simulink model "auto_pilot_upl_20240129"  (R2022b)
settings: Solver=FixedStepAuto  StartTime=0.0  StopTime=Inf  FixedStep=0.001  RelTol=1e-3  EnableMultiTasking=on
InitFcn:
  | clear mex
model workspace (MAT data in the model file):
  worldsim_instance.endpoint_ip = '127.0.0.1'
  worldsim_instance.endpoint_port = 8080
values from neighbouring files (symbols this model uses):
  ACC_Adaptive_D = 0    [AutoPilot_parameters.m]    (also in ap_ini_param.mat; ap_initialModel.sldd = 0.0)
  ACC_Adaptive_I = 0    [AutoPilot_parameters.m]    (also in ap_ini_param.mat; ap_initialModel.sldd = 0.0)
  ACC_Adaptive_P = [5 7.5]    [AutoPilot_parameters.m]    (also in ap_ini_param.mat; ap_initialModel.sldd = 5.0 7.5)
  ACC_Classic_I = 5    [AutoPilot_parameters.m]    (also in ap_ini_param.mat; ap_initialModel.sldd = 5.0)
  ACC_Classic_P = 15    [AutoPilot_parameters.m]    (also in ap_ini_param.mat; ap_initialModel.sldd = 15.0)
  ACC_MaxBrake = 50    [AutoPilot_parameters.m]    (also in ap_ini_param.mat; ap_initialModel.sldd = 50.0)
  ACC_MaxThrottle = 130    [AutoPilot_parameters.m]    (also in ap_ini_param.mat = 80; ap_initialModel.sldd = 130.0)
  ACC_Module_Activity_Flag = 1    [AutoPilot_parameters.m]    (also in ap_ini_param.mat; ap_initialModel.sldd = 1.0)
  ACC_Ready_Speed = 30    [AutoPilot_parameters.m]    (also in ap_ini_param.mat; ap_initialModel.sldd = 30.0)
  ACC_SensorMaxDistance = 250    [AutoPilot_parameters.m]    (also in ap_ini_param.mat = 120; ap_initialModel.sldd = 250.0)
  ACC_Speed_Distance_control = 3    [AutoPilot_parameters.m]    (also in ap_ini_param.mat; ap_initialModel.sldd = 3.0)
  ACC_Speed_Distance_Gain = [0.1 0.15 0.2 0.25]    [AutoPilot_parameters.m]    (also in ap_ini_param.mat; ap_initialModel.sldd = 0.1 0.15 0.2 0.25)
  ADAS_Control_Mode = 1    [AutoPilot_parameters.m]    (also in ap_ini_param.mat; ap_initialModel.sldd = 1.0)
  AEB_Alarm_Freq = 5    [AutoPilot_parameters.m]    (also in ap_ini_param.mat; ap_initialModel.sldd = 5.0)
  AEB_Distance_To_Collision_Brake = 5    [AutoPilot_parameters.m]    (also in ap_ini_param.mat; ap_initialModel.sldd = 5.0)
  AEB_Freq_Hz = Sensor_Freq_worldsim/2    (= 25)    [AutoPilot_parameters.m]    (also in ap_ini_param.mat; ap_initialModel.sldd = 25.0)
  AEB_Gain = [1 1]    [AutoPilot_parameters.m]    (also in ap_ini_param.mat; ap_initialModel.sldd = 1.0 1.0)
  AEB_Gain_set = 60    [AutoPilot_parameters.m]    (also in ap_ini_param.mat; ap_initialModel.sldd = 60.0)
  AEB_Gain_set_mult = 0.03    [AutoPilot_parameters.m]    (also in ap_ini_param.mat; ap_initialModel.sldd)
  AEB_Max_Decel = [8 15]    [AutoPilot_parameters.m]    (also in ap_ini_param.mat; ap_initialModel.sldd = 8.0 15.0)
  AEB_Max_Speed = 150    [AutoPilot_parameters.m]    (also in ap_ini_param.mat = 100; ap_initialModel.sldd = 150.0)
  AEB_Min_Distance_at_Stop = 1    [AutoPilot_parameters.m]    (also in ap_ini_param.mat; ap_initialModel.sldd = 1.0)
  AEB_Module_Activity_Flag = 1    [AutoPilot_parameters.m]    (also in ap_ini_param.mat; ap_initialModel.sldd = 1.0)
  AEB_Pedestrian_type = 68    [AutoPilot_parameters.m]    (also in ap_ini_param.mat; ap_initialModel.sldd = 68.0)
  AEB_Steer_Max = 180    [AutoPilot_parameters.m]    (also in ap_ini_param.mat; ap_initialModel.sldd = 180.0)
  AP_Activity_Flag = 1    [AutoPilot_parameters.m]    (also in ap_ini_param.mat; ap_initialModel.sldd = 1.0)
  AP_D = [0.3 0.3]    [AutoPilot_parameters.m]    (also in ap_ini_param.mat; ap_initialModel.sldd = 0.3 0.3)
  AP_Dyn_Rate_Limiter_Gain = 0.1    [AutoPilot_parameters.m]    (also in ap_ini_param.mat; ap_initialModel.sldd)
  AP_Dyn_Rate_Limiter_Power = 10    [AutoPilot_parameters.m]    (also in ap_ini_param.mat; ap_initialModel.sldd = 10.0)
  AP_Error_Max = 3    [AutoPilot_parameters.m]    (also in ap_ini_param.mat; ap_initialModel.sldd = 3.0)
  AP_Freq_Hz = Sensor_Freq_worldsim    (= 50)    [AutoPilot_parameters.m]    (also in ap_ini_param.mat; ap_initialModel.sldd = 50.0)
  AP_I = [0.05 0.05]    [AutoPilot_parameters.m]    (also in ap_ini_param.mat; ap_initialModel.sldd = 0.05 0.05)
  AP_Max_Error_dydt_Disable = 0.5    [AutoPilot_parameters.m]    (also in ap_ini_param.mat; ap_initialModel.sldd)
  AP_On_Request_Time = 0.01    [AutoPilot_parameters.m]    (also in ap_ini_param.mat; ap_initialModel.sldd)
  AP_P = [0.2 0.2]    [AutoPilot_parameters.m]    (also in ap_ini_param.mat; ap_initialModel.sldd = 0.2 0.2)
  AP_Steer_Error_Max = 0.7    [AutoPilot_parameters.m]    (also in ap_ini_param.mat; ap_initialModel.sldd)
  AP_Steer_Rate_Max_radps = 1    [AutoPilot_parameters.m]    (also in ap_ini_param.mat; ap_initialModel.sldd = 1.0)
  AP_Transition_Rate = 0.5    [AutoPilot_parameters.m]    (also in ap_ini_param.mat; ap_initialModel.sldd)
  butter_a = [1 -1.9911142922 0.991153595869]    [ap_ini_param.mat]    (also in ap_initialModel.sldd = 1.0 -1.9911142922016536 0.99115359586893548)
  butter_b = [9.82591682048e-06 1.9651833641e-05 9.82591682048e-06]    [ap_ini_param.mat]    (also in ap_initialModel.sldd = 9.825916820482009E-6 1.9651833640964018E-5 9.825916820482009)
  Lane_Width = 3.7    [AutoPilot_parameters.m]    (also in ap_ini_param.mat; ap_initialModel.sldd)
  No_Target_Display_Value = 0    [AutoPilot_parameters.m]    (also in ap_ini_param.mat; ap_initialModel.sldd = 0.0)
  radar_source = 2    [AutoPilot_parameters.m]    (also in ap_ini_param.mat; ap_initialModel.sldd = 2.0)
  Sensor_Freq_worldsim = 50    [AutoPilot_parameters.m]    (also in ap_ini_param.mat; ap_initialModel.sldd = 50.0; launcher.m)
  stop_number_collisions = 10.0    [ap_initialModel.sldd]    (also in launcher.m = 10)
  stop_speed = 0.001    [ap_initialModel.sldd]    (also in launcher.m)
  stop_time = 12.0    [ap_initialModel.sldd]    (also in launcher.m = 12)
  vehicle_width = 2.2    [AutoPilot_parameters.m]    (also in ap_ini_param.mat = 1.86; ap_initialModel.sldd)
undefined symbols (not defined in the file or in its folder): blockPlatform, light_brake_center, light_brake_left, light_brake_right
libraries: simulink x82, simwbSfunlib x32, viworldsim_lib x5, slpidlib x4, simwbUDPBlocklib x1
(part 1 of 4)
settings Model: Creator=mcava  LastModifiedBy=pumpaipa
settings SolverCC: AlgebraicLoopSolver=TrustRegion  AutoInsertRateTranBlk=on
settings DataIOCC: LimitDataPoints=on  SaveFormat=Array  ReturnWorkspaceOutputs=off  SignalLoggingName=sigsOut
settings OptimizationCC: ExpressionDepthLimit=2147483647  InitFltsAndDblsToZero=on
settings DebuggingCC: SignalInfNanChecking=warning  UnderspecifiedInitializationDetection=Classic  MergeDetectMultiDrivingBlocksExec=none  SignalResolutionControl=TryResolveAllWithWarning  MultiTaskDSMMsg=warning  MultiTaskCondExecSysMsg=none  FcnCallInpInsideContextMsg=warning  UnconnectedInputMsg=warning  UnconnectedOutputMsg=warning  UnconnectedLineMsg=warning  StateNameClashWarn=warning  SFUnexpectedBacktrackingDiag=warning  SFNoUnconditionalDefaultTransitionDiag=warning  SFExecutionAtInitializationDiag=none  SFMachineParentedDataDiag=warning  ArithmeticOperatorsInVariantConditions=warning
settings HardwareCC: ProdBitPerLong=64  ProdHWDeviceType=Intel->x86-64 (Linux 64)  TargetHWDeviceType=32-bit Generic
settings ModelReferenceCC: EnableRefExpFcnMdlSchedulingChecks=on  PropagateSignalLabelsOutOfModel=off
settings SFSimCC: SimUseLocalCustomCode=off  CustomCodeUndefinedFunction=UseInterfaceOnly
settings RTWCC: Description=VI-CarRealTime Solver Plugin V1.0  SystemTargetFile=vicrt_plugin.tlc  GenCodeOnly=on  PackageGeneratedCodeAndArtifacts=on  TemplateMakefile=vicrt_plugin_ccur.tmf  PostCodeGenCommand=if strcmp(get_param(bdroot,'TemplateMakefile'),'vicrt_plugin_ccur.tmf'),copyfile([matlabroot,filesep,'rtw',filesep,'c',filesep,'tools',filesep,'unixtools.mk'],'unixtools.mk'),if ~verLessThan('matlab','9.6'),set_param(bdroot,'MatFileLogging','off'),end,end  RTWUseLocalCustomCode=off
settings CodeAppCC: MaxIdLength=80  StateflowObjectComments=on
settings STFCustomTargetCC: ModelReferenceCompliant=off  CombineOutputUpdateFcns=on  SystemTargetFile=vicrt_plugin.tlc
settings GRTTargetCC: TargetLangStandard=C89/C90 (ANSI)  ModelReferenceCompliant=off  ParMdlRefBuildCompliant=off  CompOptLevelCompliant=off  ConcurrentExecutionCompliant=off  MatFileLogging=off  CPPClassGenCompliant=off  UseToolchainInfoCompliant=off  RTWCAPIParams=on
settings ConfigComp: CovMetricSettings=dw  CovSaveCumulativeToWorkspaceVar=on  CovSaveSingleToWorkspaceVar=on  CovExternalEMLEnable=off

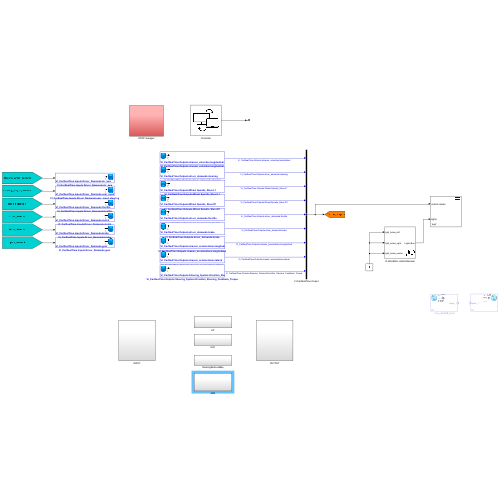
[thumbnail: Simulink's stored preview of the top-level diagram]
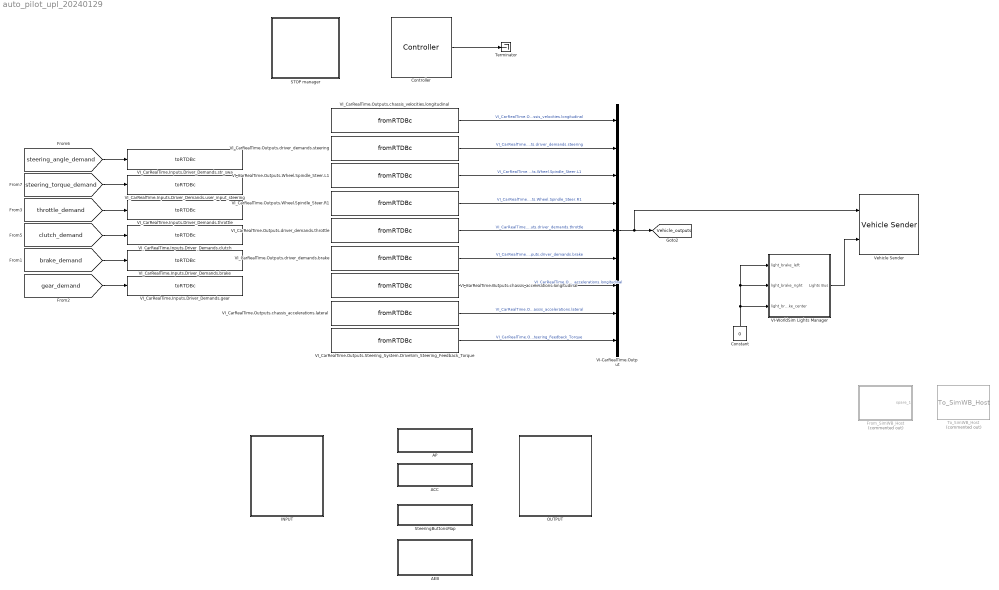
== system auto_pilot_upl_20240129 ==
  ACC : Subsystem
  AEB : Subsystem
  AP : Subsystem
  Constant : Constant  Value=0
  Controller : viworldsim_lib/Controller  worldsim_endpoint_ip=worldsim_instance.endpoint_ip  worldsim_endpoint_port=worldsim_instance.endpoint_port  worldsim_verbose=off
  From_SimWB_Host : Subsystem  Commented=on  mask(From_SimWB_Host){numPorts=1, inheritPortNames=off, portNames={'spare_1'}, origNumPorts=1, blockCode=6578738372in, localIP='255.255.255.255', localPort=25000, remoteURL='0.0.0.0', recvBufferSize=8, dims=8, blockingTime=0.01, sampletime=0.01, signalDatatype=uint8, isVarSize=off, blockPlatform=blockPlatform, msk_dimensions={1}, msk_datatypes={'double'}, byteAlign=1}
      mask prompts: numPorts "Number of Ports:"; inheritPortNames "Inherit Port Names:"; portNames "Port Names: {'a','b','c'}"; origNumPorts "Orig Num"; blockCode "Block Code"; localIP "Local IP address (SimWB sends data to this IP)"; localPort "Local IP port:"; remoteURL "Remote IP address ('0.0.0.0' to accept all):"; recvBufferSize "Receive buffer size (bytes):"; dims "Maximum length for Message:"; blockingTime "Blocking time (seconds):"; sampletime "Sample time (seconds):"; signalDatatype "Data type for Message:"; isVarSize "Output variable-size signal"; blockPlatform "Block Platform:"; msk_dimensions "Output port dimensions:"; msk_datatypes "Output port data type:"; byteAlign "Byte alignment:"
      mask help: This block receives UDP packets from the specified SimWB host. This block is supported in MATLAB R2011a and later only.
      mask init:
      | set_param(gcbh,'blockCode','6578738372in');
      mask Help: web([simwbroot 'html' filesep 'simwb_blocks_udp.html'])
      mask Callback numPorts: UDPBlockSetup(gcbh,'INPUT');
      mask Callback inheritPortNames:
      | maskVisibilities =  get_param(gcbh,'MaskVisibilities');
      | if  strcmp(get_param(gcbh,'inheritPortNames'),'on')
      |     maskVisibilities{3} = 'off';
      | else
      |     maskVisibilities{3} = 'on';
      | end
      | set_param(gcbh,'MaskVisibilities',maskVisibilities);
      mask Callback portNames: UDPBlockSetup(gcbh,'UPDATEOUTPORTNAMES');
      mask Callback msk_dimensions: UDPBlockSetup(gcbh,'BYTEUNPACKCHANGED');
      mask Callback msk_datatypes: UDPBlockSetup(gcbh,'BYTEUNPACKCHANGED');
      mask Display: image(imread('udpreceive.png'),'top-left')
  INPUT : Subsystem
  OUTPUT : Subsystem
  STOP manager : Subsystem
  SteeringButtonsMap : Subsystem
  Terminator : Terminator
  To_SimWB_Host : simwbUDPBlocklib/To_SimWB_Host  Commented=on  numPorts=1  inheritPortNames=off  portNames={'spare_1'}  remoteURL='255.255.255.255'  remotePort=25000  blockPlatform=HOST  msk_datatypes={'double'}  byteAlign=1  origNumPorts=1  blockCode=6578738372out
      settings: SourceProductName=SimWB MLToolkit
  VI-CarRealTime.Output : BusCreator  Inputs=9
  VI-WorldSim Lights Manager : Subsystem  mask{DummyMaskPar=0}
      mask init:
      | set_param(gcb, 'LinkStatus','none')
      settings: OpenFcn=|
      | wsoffline_lightsmanager;
      | set_param(gcb, 'LinkStatus','none');
      mask Display:
      | color('black');
      | image('lights.png', [85 0 50 50]);
  VI_CarRealTime.Inputs.Driver_Demands.brake : simwbSfunlib/toRTDBc  stringBlock=off  varName=VI_CarRealTime.Inputs.Driver_Demands.brake  sigDim=[1 1]  sigType=double  sampleTime=[-1 0]  maxBuffSize=1024  busName=nobus  defaultValue=0  defaultString=simwbout  hasMapping=0  ptrName=VI_CarRealTime_Inputs_Driver_Demands_brake  enumOrAlias=nothing
      settings: SourceProductName=SimWB MLToolkit
  VI_CarRealTime.Inputs.Driver_Demands.clutch : simwbSfunlib/toRTDBc  stringBlock=off  varName=VI_CarRealTime.Inputs.Driver_Demands.clutch  sigDim=[1 1]  sigType=double  sampleTime=[-1 0]  maxBuffSize=1024  busName=nobus  defaultValue=0  defaultString=simwbout  hasMapping=0  ptrName=VI_CarRealTime_Inputs_Driver_Demands_clutch  enumOrAlias=nothing
      settings: SourceProductName=SimWB MLToolkit
  VI_CarRealTime.Inputs.Driver_Demands.gear : simwbSfunlib/toRTDBc  stringBlock=off  varName=VI_CarRealTime.Inputs.Driver_Demands.gear  sigDim=[1 1]  sigType=double  sampleTime=[-1 0]  maxBuffSize=1024  busName=nobus  defaultValue=0  defaultString=simwbout  hasMapping=0  ptrName=VI_CarRealTime_Inputs_Driver_Demands_gear  enumOrAlias=nothing
      settings: SourceProductName=SimWB MLToolkit
  VI_CarRealTime.Inputs.Driver_Demands.str_swa : simwbSfunlib/toRTDBc  stringBlock=off  varName=VI_CarRealTime.Inputs.Driver_Demands.str_swa  sigDim=[1 1]  sigType=double  sampleTime=[-1 0]  maxBuffSize=1024  busName=nobus  defaultValue=0  defaultString=simwbout  hasMapping=0  ptrName=VI_CarRealTime_Inputs_Driver_Demands_str_swa  enumOrAlias=nothing
      settings: SourceProductName=SimWB MLToolkit
  VI_CarRealTime.Inputs.Driver_Demands.throttle : simwbSfunlib/toRTDBc  stringBlock=off  varName=VI_CarRealTime.Inputs.Driver_Demands.throttle  sigDim=[1 1]  sigType=double  sampleTime=[-1 0]  maxBuffSize=1024  busName=nobus  defaultValue=0  defaultString=simwbout  hasMapping=0  ptrName=VI_CarRealTime_Inputs_Driver_Demands_throttle  enumOrAlias=nothing
      settings: SourceProductName=SimWB MLToolkit
  VI_CarRealTime.Inputs.Driver_Demands.user_input_steering : simwbSfunlib/toRTDBc  stringBlock=off  varName=VI_CarRealTime.Inputs.Driver_Demands.user_input_steering  sigDim=[1 1]  sigType=double  sampleTime=[-1 0]  maxBuffSize=1024  busName=nobus  defaultValue=0  defaultString=simwbout  hasMapping=0  ptrName=VI_CarRealTime_Inputs_Driver_Demands_user_input_steering  enumOrAlias=nothing
      settings: SourceProductName=SimWB MLToolkit
  VI_CarRealTime.Outputs.Steering_System.DriveSim_Steering_Feedback_Torque : simwbSfunlib/fromRTDBc  stringBlock=off  varName=VI_CarRealTime.Outputs.Steering_System.DriveSim_Steering_Feedback_Torque  sigDim=[1 1]  sigType=double  sampleTime=[-1 0]  maxBuffSize=1024  busName=nobus  defaultValue=0  defaultString=simwbin  hasMapping=0  ptrName=VI_CarRealTime_Outputs_Steering_System_DriveSim_Steering_Feedback_Torque  enumOrAlias=nothing
      settings: SourceProductName=SimWB MLToolkit
  VI_CarRealTime.Outputs.Wheel.Spindle_Steer.L1 : simwbSfunlib/fromRTDBc  stringBlock=off  varName=VI_CarRealTime.Outputs.Wheel.Spindle_Steer.L1  sigDim=[1 1]  sigType=double  sampleTime=[-1 0]  maxBuffSize=1024  busName=nobus  defaultValue=0  defaultString=simwbin  hasMapping=0  ptrName=VI_CarRealTime_Outputs_Wheel_Spindle_Steer_L1  enumOrAlias=nothing
      settings: SourceProductName=SimWB MLToolkit
  VI_CarRealTime.Outputs.Wheel.Spindle_Steer.R1 : simwbSfunlib/fromRTDBc  stringBlock=off  varName=VI_CarRealTime.Outputs.Wheel.Spindle_Steer.R1  sigDim=[1 1]  sigType=double  sampleTime=[-1 0]  maxBuffSize=1024  busName=nobus  defaultValue=0  defaultString=simwbin  hasMapping=0  ptrName=VI_CarRealTime_Outputs_Wheel_Spindle_Steer_R1  enumOrAlias=nothing
      settings: SourceProductName=SimWB MLToolkit
  VI_CarRealTime.Outputs.chassis_accelerations.lateral : simwbSfunlib/fromRTDBc  stringBlock=off  varName=VI_CarRealTime.Outputs.chassis_accelerations.lateral  sigDim=[1 1]  sigType=double  sampleTime=[-1 0]  maxBuffSize=1024  busName=nobus  defaultValue=0  defaultString=simwbin  hasMapping=0  ptrName=VI_CarRealTime_Outputs_chassis_accelerations_lateral  enumOrAlias=nothing
      settings: SourceProductName=SimWB MLToolkit
  VI_CarRealTime.Outputs.chassis_accelerations.longitudinal : simwbSfunlib/fromRTDBc  stringBlock=off  varName=VI_CarRealTime.Outputs.chassis_accelerations.longitudinal  sigDim=[1 1]  sigType=double  sampleTime=[-1 0]  maxBuffSize=1024  busName=nobus  defaultValue=0  defaultString=simwbin  hasMapping=0  ptrName=VI_CarRealTime_Outputs_chassis_accelerations_longitudinal  enumOrAlias=nothing
      settings: SourceProductName=SimWB MLToolkit
  VI_CarRealTime.Outputs.chassis_velocities.longitudinal : simwbSfunlib/fromRTDBc  stringBlock=off  varName=VI_CarRealTime.Outputs.chassis_velocities.longitudinal  sigDim=[1 1]  sigType=double  sampleTime=[-1 0]  maxBuffSize=1024  busName=nobus  defaultValue=0  defaultString=simwbin  hasMapping=0  ptrName=VI_CarRealTime_Outputs_chassis_velocities_longitudinal  enumOrAlias=nothing
      settings: SourceProductName=SimWB MLToolkit
  VI_CarRealTime.Outputs.driver_demands.brake : simwbSfunlib/fromRTDBc  stringBlock=off  varName=VI_CarRealTime.Outputs.driver_demands.brake  sigDim=[1 1]  sigType=double  sampleTime=[-1 0]  maxBuffSize=1024  busName=nobus  defaultValue=0  defaultString=simwbin  hasMapping=0  ptrName=VI_CarRealTime_Outputs_driver_demands_brake  enumOrAlias=nothing
      settings: SourceProductName=SimWB MLToolkit
  VI_CarRealTime.Outputs.driver_demands.steering : simwbSfunlib/fromRTDBc  stringBlock=off  varName=VI_CarRealTime.Outputs.driver_demands.steering  sigDim=[1 1]  sigType=double  sampleTime=[-1 0]  maxBuffSize=1024  busName=nobus  defaultValue=0  defaultString=simwbin  hasMapping=0  ptrName=VI_CarRealTime_Outputs_driver_demands_steering  enumOrAlias=nothing
      settings: SourceProductName=SimWB MLToolkit
  VI_CarRealTime.Outputs.driver_demands.throttle : simwbSfunlib/fromRTDBc  stringBlock=off  varName=VI_CarRealTime.Outputs.driver_demands.throttle  sigDim=[1 1]  sigType=double  sampleTime=[-1 0]  maxBuffSize=1024  busName=nobus  defaultValue=0  defaultString=simwbin  hasMapping=0  ptrName=VI_CarRealTime_Outputs_driver_demands_throttle  enumOrAlias=nothing
      settings: SourceProductName=SimWB MLToolkit
  Vehicle Sender : viworldsim_lib/VI-WorldSim Vehicle Senders/Vehicle Sender  useOutputMapInMaskFlag=on  worldsim_car_name='ego'  worldsim_ai_controlled=off
      link override VI_WorldSim_VehicleSender: worldsim_car_name='ego'
  tag scope: Vehicle_outputs=global
  wires:
  [throttle_demand] -> VI_CarRealTime.Inputs.Driver_Demands.throttle/1
  [clutch_demand] -> VI_CarRealTime.Inputs.Driver_Demands.clutch/1
  [steering_angle_demand] -> VI_CarRealTime.Inputs.Driver_Demands.str_swa/1
  [steering_torque_demand] -> VI_CarRealTime.Inputs.Driver_Demands.user_input_steering/1
  [brake_demand] -> VI_CarRealTime.Inputs.Driver_Demands.brake/1
  [gear_demand] -> VI_CarRealTime.Inputs.Driver_Demands.gear/1
  Controller/1 -> Terminator/1
  Constant/1 -> VI-WorldSim Lights Manager/3(light_brake_center), VI-WorldSim Lights Manager/2(light_brake_right), VI-WorldSim Lights Manager/1(light_brake_left)
  VI-WorldSim Lights Manager/1(Lights Bus) -> Vehicle Sender/2
  VI_CarRealTime.Outputs.chassis_velocities.longitudinal/1 -> VI-CarRealTime.Output/1  "VI_CarRealTime.Outputs.chassis_velocities.longitudinal"
  VI_CarRealTime.Outputs.driver_demands.steering/1 -> VI-CarRealTime.Output/2  "VI_CarRealTime.Outputs.driver_demands.steering"
  VI_CarRealTime.Outputs.Wheel.Spindle_Steer.L1/1 -> VI-CarRealTime.Output/3  "VI_CarRealTime.Outputs.Wheel.Spindle_Steer.L1"
  VI_CarRealTime.Outputs.Wheel.Spindle_Steer.R1/1 -> VI-CarRealTime.Output/4  "VI_CarRealTime.Outputs.Wheel.Spindle_Steer.R1"
  VI_CarRealTime.Outputs.driver_demands.brake/1 -> VI-CarRealTime.Output/6  "VI_CarRealTime.Outputs.driver_demands.brake"
  VI_CarRealTime.Outputs.driver_demands.throttle/1 -> VI-CarRealTime.Output/5  "VI_CarRealTime.Outputs.driver_demands.throttle"
  VI_CarRealTime.Outputs.chassis_accelerations.longitudinal/1 -> VI-CarRealTime.Output/7  "VI_CarRealTime.Outputs.chassis_accelerations.longitudinal"
  VI_CarRealTime.Outputs.chassis_accelerations.lateral/1 -> VI-CarRealTime.Output/8  "VI_CarRealTime.Outputs.chassis_accelerations.lateral"
  VI_CarRealTime.Outputs.Steering_System.DriveSim_Steering_Feedback_Torque/1 -> VI-CarRealTime.Output/9  "VI_CarRealTime.Outputs.Steering_System.DriveSim_Steering_Feedback_Torque"
  VI-CarRealTime.Output/1 -> Vehicle Sender/1, [Vehicle_outputs]

== system auto_pilot_upl_20240129/ACC ==
  ACC_Inputs : Subsystem
  ACC_Logic : Subsystem
  ACC_Outputs : Subsystem

== system auto_pilot_upl_20240129/AEB ==
  AEB_Inputs : Subsystem
  AEB_Logic : Subsystem
  AEB_Outputs : Subsystem

== system auto_pilot_upl_20240129/AP ==
  AP_Inputs : Subsystem
  AP_Logic : Subsystem
  AP_Outputs : Subsystem

== system auto_pilot_upl_20240129/From_SimWB_Host ==
  Byte Unpack : S-Function  FunctionName=byte2any  Parameters=dimensionsout, datatypesout, byteAlign  SFunctionDeploymentMode=off  EnableBusSupport=off  mask(Byte Unpack){dimensions={1}, datatypes={'double'}, byteAlign=1}
      mask prompts: dimensions "Output port dimensions (cell array):"; datatypes "Output port data types (cell array):"; byteAlign "Byte alignment:"
      mask help: Unpack a binary byte vector to extract data. Insert after a UDP Recv block to break-up a UDP packet into its constituent data vectors.
      mask init:
      | [dimensionsout, datatypesout]= byteunpack_callback(dimensions, datatypes);
      mask Help: eval('linkfoundation.util.blockHelpLink(''ecoder'')');
      mask TypeOptions byteAlign: 1 | 2 | 4 | 8
      mask Display:
      | color('blue');
      | text(0.95, 0.90, '', ...
      |                 'horizontalalignment', 'right');
      | color('black');
      | text(0.50, 0.12, 'Byte Unpack', ...
      |                 'horizontalAlignment','center');
  Term : Terminator
  UDP Receive : S-Function  FunctionName=sdspFromNetwork  Parameters=localURL, localPort, remoteURL, remotePort, recvBufferSize, signalDatatype, dims, sampletime, isVarSize, blockingTime  SFunctionDeploymentMode=off  EnableBusSupport=off  mask(UDP Receive){localURL='0.0.0.0', localPort=localPort, remoteURL=remoteURL, remotePort=-1, recvBufferSize=recvBufferSize, dims=dims, signalDatatype=uint8, isVarSize=off, showBlockingTime=on, blockingTime=blockingTime, sampletime=sampletime, blockPlatform=blockPlatform}
      mask prompts: localURL "Local IP address:"; localPort "Local IP port:"; remoteURL "Remote IP address ('0.0.0.0' to accept all):"; remotePort "Remote IP port:"; recvBufferSize "Receive buffer size (bytes):"; dims "Maximum length for Message:"; signalDatatype "Data type for Message:"; isVarSize "Output variable-size signal"; showBlockingTime "Show blocking time"; blockingTime "Blocking time (seconds):"; sampletime "Sample time (seconds):"; blockPlatform "Block Platform"
      mask help:
      | Receive UDP packets on a given IP port.
      | This block receives a UDP packet from the network and emits that data as a one-dimensional vector of the specified data type.
      mask init:
      | icon = sprintf('%s\n', 'fprintf(''UDP Receive'');');
      | % If there are multiple ports, label them
      | if strcmp(get_param(gcb,'isVarSize'), 'off')
      |     icon = sprintf('%s%s\n', icon, 'port_label(''output'', 1, ''Message'');');
      |     icon = sprintf('%s%s\n', icon, 'port_label(''output'', 2, ''Length'');');
      | end
      | icon = [icon sprintf('%s\n','color(''blue'');')];
      | icon = [icon sprintf('%s\n','text(0.97, 0.87, get_param(gcb, ''blockPlatform''), ''horizontalalignment'', ''right'');')];
      | set_param(gcb, 'maskDisplay', icon);
      | 
      | % Hide the lengthDatatype and BlockingTime if required
      | vis = get_param(gcbh, 'MaskVisibilities');
      | vis{10} = get_param(gcbh, 'showBlockingTime');
      | set_param(gcbh, 'MaskVisibilities', vis);
      mask Help: eval('dspnetwork_help(''UDPReceive'')')
      mask TypeOptions signalDatatype: double | single | int8 | uint8 | int16 | uint16 | int32 | uint32 | boolean
      mask Display:
      | fprintf('UDP Receive');
      | port_label('output', 1, 'Message');
      | port_label('output', 2, 'Length');
      | color('blue');
      | text(0.97, 0.87, get_param(gcb, 'blockPlatform'), 'horizontalalignment', 'right');
  spare_1 : Outport
  wires:
  UDP Receive/2 -> Term/1
  UDP Receive/1 -> Byte Unpack/1
  Byte Unpack/1 -> spare_1/1

== system auto_pilot_upl_20240129/INPUT ==
  Inputs for CRT : Subsystem

== system auto_pilot_upl_20240129/OUTPUT ==
  VI-CarRealTime_Outputs : Subsystem
  VI-CarRealTime_Outputs2 : Subsystem  Commented=on
  WorldSim_Sensor_Outputs : Subsystem
  rough data reporting : Subsystem

== system auto_pilot_upl_20240129/STOP manager ==
  Clock2 : Clock
  Compare To Constant : simulink/Logic and Bit Operations/Compare To Constant  relop=>  const=stop_time  OutDataTypeStr=boolean
  Compare To Constant1 : simulink/Logic and Bit Operations/Compare To Constant  relop=<=  const=stop_speed  OutDataTypeStr=boolean
  Compare To Constant2 : simulink/Logic and Bit Operations/Compare To Constant  relop=>=  const=stop_number_collisions  OutDataTypeStr=boolean
  Constant : Constant  Value=0
  OR : Logic  Operator=OR  Inputs=4  AllPortsSameDT=off  OutDataTypeStr=boolean
  Stop Simulation : Stop
  wires:
  [collision_additive] -> Compare To Constant2/1
  Compare To Constant2/1 -> OR/3
  Compare To Constant/1 -> OR/1
  [Vehicle_Speed] -> Compare To Constant1/1
  Clock2/1 -> Compare To Constant/1
  Compare To Constant1/1 -> OR/2
  OR/1 -> Stop Simulation/1
  [LKA_Stop_signal] -> OR/4
  Constant/1 -> [LKA_Stop_signal]

== system auto_pilot_upl_20240129/SteeringButtonsMap ==
  VI_DriveSim.Inputs.Control.VICRT_RESTART_REQ : simwbSfunlib/toRTDBc  stringBlock=off  varName=VI_DriveSim.Inputs.Control.VICRT_RESTART_REQ  sigDim=[1 1]  sigType=double  sampleTime=[-1 0]  maxBuffSize=1024  busName=nobus  defaultValue=0  defaultString=simwbout  hasMapping=0  ptrName=VI_DriveSim_Inputs_ECAT_BECKH_DIG4  enumOrAlias=nothing
      settings: SourceProductName=SimWB MLToolkit
  VI_DriveSim.Inputs.Control.VICRT_RESTORE_REQ : simwbSfunlib/toRTDBc  stringBlock=off  varName=VI_DriveSim.Inputs.Control.VICRT_RESTORE_REQ  sigDim=[1 1]  sigType=double  sampleTime=[-1 0]  maxBuffSize=1024  busName=nobus  defaultValue=0  defaultString=simwbout  hasMapping=0  ptrName=VI_DriveSim_Inputs_ECAT_BECKH_DIG3  enumOrAlias=nothing
      settings: SourceProductName=SimWB MLToolkit
  VI_DriveSim.Inputs.ECAT.BECKH.DIG3 : simwbSfunlib/fromRTDBc  stringBlock=off  varName=VI_DriveSim.Inputs.ECAT.BECKH.DIG3  sigDim=[1 1]  sigType=double  sampleTime=[-1 0]  maxBuffSize=1024  busName=nobus  defaultValue=0  defaultString=simwbin  hasMapping=0  ptrName=varName  enumOrAlias=nothing
      settings: SourceProductName=SimWB MLToolkit
  VI_DriveSim.Inputs.ECAT.BECKH.DIG4 : simwbSfunlib/fromRTDBc  stringBlock=off  varName=VI_DriveSim.Inputs.ECAT.BECKH.DIG4  sigDim=[1 1]  sigType=double  sampleTime=[-1 0]  maxBuffSize=1024  busName=nobus  defaultValue=0  defaultString=simwbin  hasMapping=0  ptrName=VI_DriveSim_Inputs_ECAT_BECKH_DIG4  enumOrAlias=nothing
      settings: SourceProductName=SimWB MLToolkit
  wires:
  VI_DriveSim.Inputs.ECAT.BECKH.DIG3/1 -> VI_DriveSim.Inputs.Control.VICRT_RESTORE_REQ/1
  VI_DriveSim.Inputs.ECAT.BECKH.DIG4/1 -> VI_DriveSim.Inputs.Control.VICRT_RESTART_REQ/1

== system auto_pilot_upl_20240129/VI-WorldSim Lights Manager ==
  light_brake_left : Inport
  light_brake_right : Inport  Port=2
  light_brake_center : Inport  Port=3
  Lights : Subsystem
  Lights Bus : Outport  VectorParamsAs1DForOutWhenUnconnected=off
  wires:
  Lights/1(Out1) -> Lights Bus/1
  light_brake_left/1 -> Lights/1(light_brake_left)
  light_brake_right/1 -> Lights/2(light_brake_right)
  light_brake_center/1 -> Lights/3(light_brake_center)

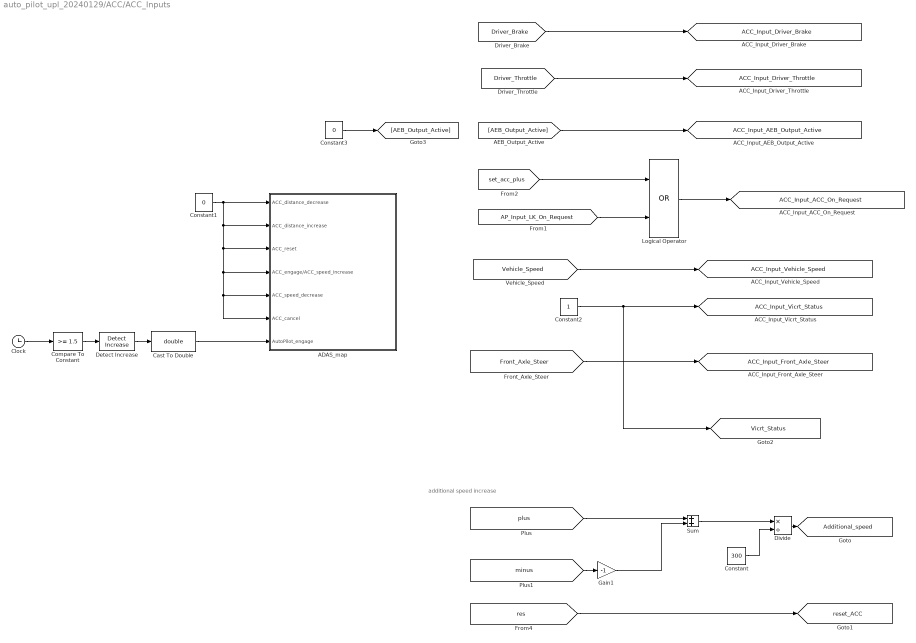
== system auto_pilot_upl_20240129/ACC/ACC_Inputs ==
  note: additional speed increase
  ADAS_map : Subsystem
  Cast To Double : DataTypeConversion  OutDataTypeStr=double  SaturateOnIntegerOverflow=off  RndMeth=Floor
  Clock : Clock
  Compare To Constant : simulink/Logic and Bit Operations/Compare To Constant  relop=>=  const=1.5  OutDataTypeStr=boolean
  Constant : Constant  Value=300
  Constant1 : Constant  Value=0
  Constant2 : Constant
  Constant3 : Constant  Value=0
  Detect Increase : simulink/Logic and Bit Operations/Detect Increase  vinit=0.0  OutDataTypeStr=boolean
  Divide : Product  Inputs=*/
  Gain1 : Gain  Gain=-1
  Logical Operator : Logic  Operator=OR  AllPortsSameDT=off  OutDataTypeStr=boolean
  Sum : Sum
  tag scope: ACC_Input_ACC_On_Request=global, ACC_Input_AEB_Output_Active=global, ACC_Input_Driver_Brake=global, ACC_Input_Driver_Throttle=global, ACC_Input_Front_Axle_Steer=global, ACC_Input_Vehicle_Speed=global, ACC_Input_Vicrt_Status=global, Additional_speed=global, Vicrt_Status=global, reset_ACC=global
  wires:
  [Driver_Brake] -> [ACC_Input_Driver_Brake]
  [Driver_Throttle] -> [ACC_Input_Driver_Throttle]
  [AEB_Output_Active] -> [ACC_Input_AEB_Output_Active]
  [Vehicle_Speed] -> [ACC_Input_Vehicle_Speed]
  Constant2/1 -> [Vicrt_Status], [ACC_Input_Vicrt_Status]
  [Front_Axle_Steer] -> [ACC_Input_Front_Axle_Steer]
  Logical Operator/1 -> [ACC_Input_ACC_On_Request]
  [plus] -> Sum/1
  [minus] -> Gain1/1
  Sum/1 -> Divide/1
  Gain1/1 -> Sum/2
  [set_acc_plus] -> Logical Operator/1
  [AP_Input_LK_On_Request] -> Logical Operator/2
  Divide/1 -> [Additional_speed]
  Constant/1 -> Divide/2
  [res] -> [reset_ACC]
  Constant1/1 -> ADAS_map/4(ACC_engage/ACC_speed_increase), ADAS_map/6(ACC_cancel), ADAS_map/5(ACC_speed_decrease), ADAS_map/3(ACC_reset), ADAS_map/2(ACC_distance_increase), ADAS_map/1(ACC_distance_decrease)
  Clock/1 -> Compare To Constant/1
  Compare To Constant/1 -> Detect Increase/1
  Detect Increase/1 -> Cast To Double/1
  Cast To Double/1 -> ADAS_map/7(AutoPilot_engage)
  Constant3/1 -> [AEB_Output_Active]

== system auto_pilot_upl_20240129/ACC/ACC_Logic ==
  ACC_Speed_Controller : Subsystem
  ACC_Switch : Subsystem
  ACC_Target_Acquisition : Subsystem

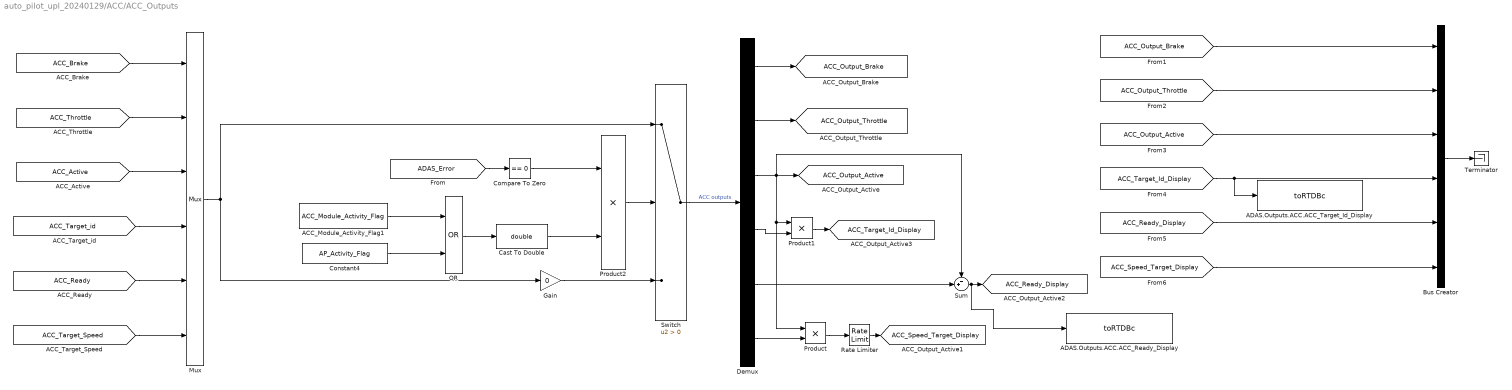
== system auto_pilot_upl_20240129/ACC/ACC_Outputs ==
  ACC_Module_Activity_Flag1 : Constant  Value=ACC_Module_Activity_Flag
  ADAS.Outputs.ACC.ACC_Ready_Display : simwbSfunlib/toRTDBc  stringBlock=off  varName=ADAS.Outputs.ACC.ACC_Ready_Display  sigDim=[1 1]  sigType=double  sampleTime=[-1 0]  maxBuffSize=1024  busName=nobus  defaultValue=0  defaultString=simwbout  hasMapping=0  ptrName=ADAS_Outputs_ACC_ACC_Target_Id_Display  enumOrAlias=nothing
      settings: SourceProductName=SimWB MLToolkit
  ADAS.Outputs.ACC.ACC_Target_Id_Display : simwbSfunlib/toRTDBc  stringBlock=off  varName=ADAS.Outputs.ACC.ACC_Target_Id_Display  sigDim=[1 1]  sigType=double  sampleTime=[-1 0]  maxBuffSize=1024  busName=nobus  defaultValue=0  defaultString=simwbout  hasMapping=0  ptrName=ADAS_Outputs_AP_AP_On  enumOrAlias=nothing
      settings: SourceProductName=SimWB MLToolkit
  Bus Creator : BusCreator  Inputs=6
  Cast To Double : DataTypeConversion  OutDataTypeStr=double  SaturateOnIntegerOverflow=off  RndMeth=Floor
  Compare To Zero : simulink/Logic and Bit Operations/Compare To Zero  relop===  OutDataTypeStr=boolean
  Constant4 : Constant  Value=AP_Activity_Flag
  Demux : Demux  Outputs=6
  Gain : Gain  Gain=0
  Mux : Mux  Inputs=6
  OR : Logic  Operator=OR  AllPortsSameDT=off  OutDataTypeStr=boolean
  Product : Product
  Product1 : Product
  Product2 : Product
  Rate Limiter : RateLimiter  RisingSlewLimit=inf  FallingSlewLimit=-100  SampleTimeMode=inherited
  Sum : Sum  Inputs=-+|
  Switch : Switch  Criteria=u2 > Threshold  SaturateOnIntegerOverflow=off  InputSameDT=off
  Terminator : Terminator
  tag scope: ACC_Output_Active=global, ACC_Output_Brake=global, ACC_Output_Throttle=global, ACC_Ready_Display=global, ACC_Speed_Target_Display=global, ACC_Target_Id_Display=global
  wires:
  [ACC_Brake] -> Mux/1
  [ACC_Throttle] -> Mux/2
  Mux/1 -> Switch/1, Gain/1
  Switch/1 -> Demux/1  "ACC outputs"
  Cast To Double/1 -> Product2/2
  Demux/1 -> [ACC_Output_Brake]
  Demux/2 -> [ACC_Output_Throttle]
  Gain/1 -> Switch/3
  [ACC_Active] -> Mux/3
  [ACC_Target_id] -> Mux/4
  Demux/4 -> Product1/2
  [ACC_Ready] -> Mux/5
  [ACC_Target_Speed] -> Mux/6
  Demux/5 -> Sum/2
  Demux/6 -> Product/2
  Product/1 -> Rate Limiter/1
  [ADAS_Error] -> Compare To Zero/1
  Product2/1 -> Switch/2
  Compare To Zero/1 -> Product2/1
  ACC_Module_Activity_Flag1/1 -> OR/1
  Constant4/1 -> OR/2
  OR/1 -> Cast To Double/1
  Demux/3 -> Sum/1, Product/1, Product1/1, [ACC_Output_Active]
  Rate Limiter/1 -> [ACC_Speed_Target_Display]
  Sum/1 -> ADAS.Outputs.ACC.ACC_Ready_Display/1, [ACC_Ready_Display]
  Product1/1 -> [ACC_Target_Id_Display]
  [ACC_Output_Brake] -> Bus Creator/1
  [ACC_Output_Throttle] -> Bus Creator/2
  [ACC_Output_Active] -> Bus Creator/3
  [ACC_Target_Id_Display] -> Bus Creator/4, ADAS.Outputs.ACC.ACC_Target_Id_Display/1
  [ACC_Ready_Display] -> Bus Creator/5
  [ACC_Speed_Target_Display] -> Bus Creator/6
  Bus Creator/1 -> Terminator/1

== system auto_pilot_upl_20240129/AEB/AEB_Inputs ==
  Gain{,1..3} (4 alike) : Gain  Gain=0
  Gain4 : Gain  Gain=-1
  Gain5 : Gain  Gain=-1
  MATLAB Function : MATLAB Function  TreatAsAtomicUnit=on
  MATLAB Function1 : MATLAB Function  TreatAsAtomicUnit=on
  Mux{,1..3} (4 alike) : Mux  Inputs=3
  tag scope: AEB_Input_Driver_Steering=global, AEB_Input_SensorTargets_azimuthInSensor_mux=global, AEB_Input_SensorTargets_distanceToCollision_mux=global, AEB_Input_SensorTargets_id_mux=global, AEB_Input_SensorTargets_type_mux=global, AEB_Input_Vehicle_Speed=global
  wires:
  [SensorTargets_300002_distanceToCollision_mux] -> MATLAB Function1/1(u)
  [SensorTargets_300001_distanceToCollision_mux] -> MATLAB Function/1(u)
  [SensorTargets_300000_distanceToCollision_mux] -> Gain/1
  [SensorTargets_300001_id_mux] -> Mux1/2
  [SensorTargets_300000_id_mux] -> Gain1/1
  [SensorTargets_300000_azimuthInSensor_mux] -> Gain2/1
  [SensorTargets_300001_azimuthInSensor_mux] -> Gain4/1
  [SensorTargets_300002_azimuthInSensor_mux] -> Gain5/1
  MATLAB Function1/1(y) -> Mux/3
  [SensorTargets_300002_id_mux] -> Mux1/3
  Gain5/1 -> Mux2/3
  [Driver_Steering] -> [AEB_Input_Driver_Steering]
  [Vehicle_Speed] -> [AEB_Input_Vehicle_Speed]
  [SensorTargets_300001_type_mux] -> Mux3/2
  [SensorTargets_300000_type_mux] -> Gain3/1
  [SensorTargets_300002_type_mux] -> Mux3/3
  Gain/1 -> Mux/1
  Gain1/1 -> Mux1/1
  Gain2/1 -> Mux2/1
  Gain3/1 -> Mux3/1
  MATLAB Function/1(y) -> Mux/2
  Gain4/1 -> Mux2/2
  Mux/1 -> [AEB_Input_SensorTargets_distanceToCollision_mux]
  Mux1/1 -> [AEB_Input_SensorTargets_id_mux]
  Mux2/1 -> [AEB_Input_SensorTargets_azimuthInSensor_mux]
  Mux3/1 -> [AEB_Input_SensorTargets_type_mux]

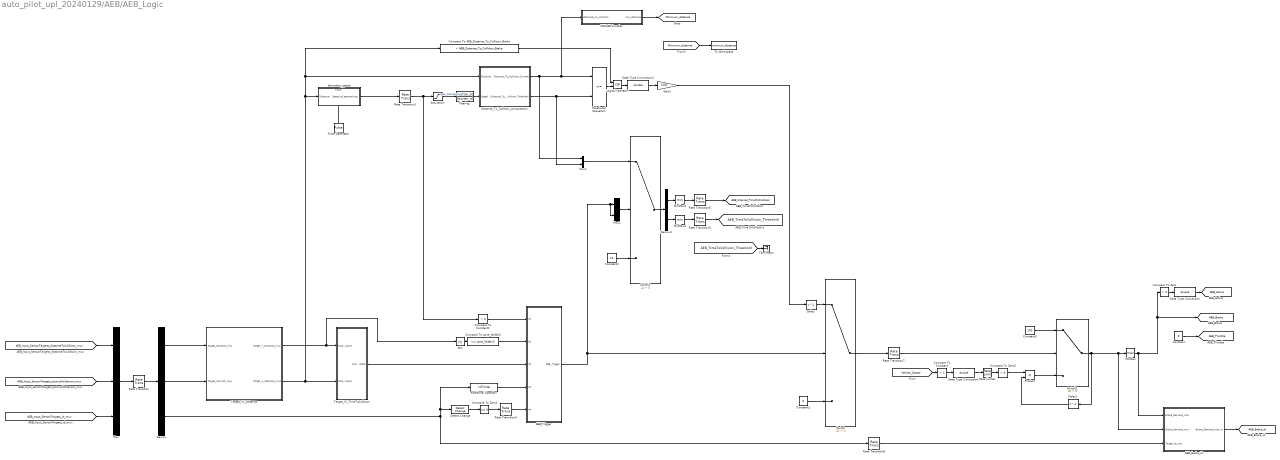
== system auto_pilot_upl_20240129/AEB/AEB_Logic ==
  "AEB_Brake_id " : Subsystem
  AEB_Trigger : Subsystem
  Abs : Abs  SaturateOnIntegerOverflow=off
  Compare To AEB_Distance_To_Collision_Brake : simulink/Logic and Bit Operations/Compare To Constant  relop=<  const=AEB_Distance_To_Collision_Brake  OutDataTypeStr=boolean
  Compare To Constant : simulink/Logic and Bit Operations/Compare To Constant  relop=>  const=1  OutDataTypeStr=boolean
  Compare To Constant1 : simulink/Logic and Bit Operations/Compare To Constant  relop=>  const=0  OutDataTypeStr=boolean
  Compare To Lane_Width/2 : simulink/Logic and Bit Operations/Compare To Constant  relop=<=  const=Lane_Width/2  OutDataTypeStr=boolean
  Compare To Zero : simulink/Logic and Bit Operations/Compare To Zero  relop=>  OutDataTypeStr=boolean
  Compare To Zero1 : simulink/Logic and Bit Operations/Compare To Zero  relop===  OutDataTypeStr=boolean
  Compare To Zero3 : simulink/Logic and Bit Operations/Compare To Zero  relop=>  OutDataTypeStr=boolean
  Constant : Constant  Value=0
  Constant1 : Constant  Value=0
  Constant2 : Constant  Value=10
  Constant3 : Constant  Value=100
  Data Type Conversion : DataTypeConversion  OutDataTypeStr=double  SaturateOnIntegerOverflow=off  RndMeth=Floor
  Data Type Conversion1 : DataTypeConversion  OutDataTypeStr=double  SaturateOnIntegerOverflow=off  RndMeth=Floor
  Data Type Conversion2 : DataTypeConversion  OutDataTypeStr=double  SaturateOnIntegerOverflow=off  RndMeth=Floor
  Delay : Delay  DelayLength=1  InitialCondition=0
  Delay1 : Delay  DelayLength=1
  Demux : Demux  Outputs=3
  Demux2 : Demux  Outputs=2
  Detect Change : simulink/Logic and Bit Operations/Detect Change  vinit=0  OutDataTypeStr=boolean
  Distance_To_Collision_computation : Subsystem
  Gain1 : Gain  Gain=100
  Logical Operator : Logic  Operator=OR  AllPortsSameDT=off  OutDataTypeStr=boolean
  MATLAB Function : MATLAB Function  TreatAsAtomicUnit=on
  MinMax : MinMax  Function=max
  MinMax3 : MinMax
  MinMax4 : MinMax
  Mux : Mux  Inputs=3
  Mux1 : Mux  Inputs=2
  Mux2 : Mux  Inputs=2
  Product : Product
  Pulse Generator : DiscretePulseGenerator  PulseType=Time based  Period=1/AEB_Freq_Hz  PulseWidth=2.5
  Rate Limiter : RateLimiter  RisingSlewLimit=inf  SampleTimeMode=inherited
  Rate Transition{,1,8..9} (4 alike) : RateTransition  OutPortSampleTime=1/AEB_Freq_Hz
  Rate Transition5 : RateTransition  OutPortSampleTime=1/1000
  Rate Transition6 : RateTransition  OutPortSampleTime=1/1000
  Rate Transition7 : RateTransition  OutPortSampleTime=1/1000
  Relational Operator : RelationalOperator  Operator=isFinite  OutDataTypeStr=boolean  InputSameDT=off
  Relational Operator1 : RelationalOperator  Operator=<=  OutDataTypeStr=boolean  InputSameDT=off
  Saturation : Saturate  UpperLimit=inf  LowerLimit=1e-6
  Switch : Switch  Criteria=u2 > Threshold  SaturateOnIntegerOverflow=off  InputSameDT=off
  Switch1 : Switch  Criteria=u2 > Threshold  SaturateOnIntegerOverflow=off  InputSameDT=off
  Switch2 : Switch  Criteria=u2 > Threshold  SaturateOnIntegerOverflow=off  InputSameDT=off
  Target_XY_Distance : MATLAB Function  TreatAsAtomicUnit=on
  Target_XY_TimeToCollision : Subsystem
  Terminator : Terminator
  To Workspace : ToWorkspace  VariableName=minimum_distance  SampleTime=-1
      settings: Save2DSignal=2-D array (concatenate along first dimension)
  derivation_speed : Subsystem
  filtering : DiscreteFilter  Numerator=[butter_b]  Denominator=[butter_a]  SampleTime=1e-3
  tag scope: AEB_Active=global, AEB_Brake=global, AEB_Brake_id=global, AEB_Internal_TimeToCollision=global, AEB_Throttle=global, AEB_TimeToCollision_Threshold=global, Minimum_distance=global
  wires:
  [AEB_Input_SensorTargets_distanceToCollision_mux] -> Mux/1
  [AEB_Input_SensorTargets_azimuthInSensor_mux] -> Mux/2
  Mux/1 -> Rate Transition/1
  Compare To Zero/1 -> Data Type Conversion/1
  [AEB_Input_SensorTargets_id_mux] -> Mux/3
  Constant1/1 -> Switch/3
  Rate Transition/1 -> Demux/1
  Switch/1 -> Rate Transition7/1
  Distance_To_Collision_computation/2(Distance_To_Collision_Threshold) -> Mux1/2, Relational Operator1/2
  Distance_To_Collision_computation/1(Distance_To_Collision_Current) -> Mux1/1, MATLAB Function/1(distances_to_collision), Relational Operator1/1
  Gain1/1 -> Delay/1
  Constant2/1 -> Switch1/3
  MinMax3/1 -> Rate Transition6/1
  Data Type Conversion1/1 -> Gain1/1
  Saturation/1 -> filtering/1  "after_saturation"
  MinMax4/1 -> Rate Transition5/1
  Mux1/1 -> Switch1/1
  Mux2/1 -> Switch1/2
  Switch1/1 -> Demux2/1
  Demux2/1 -> MinMax3/1
  Demux2/2 -> MinMax4/1
  Detect Change/1 -> Compare To Zero1/1
  "AEB_Brake_id "/1(Brake_Demand_max_id) -> [AEB_Brake_id]
  MinMax/1 -> "AEB_Brake_id "/1(Brake_Demand_max), [AEB_Brake], Compare To Zero/1
  Data Type Conversion/1 -> [AEB_Active]
  Constant/1 -> [AEB_Throttle]
  Rate Transition5/1 -> [AEB_TimeToCollision_Threshold]
  Rate Transition6/1 -> [AEB_Internal_TimeToCollision]
  Target_XY_TimeToCollision/1(Collision_Identifier) -> AEB_Trigger/3(In2)
  Compare To Zero1/1 -> Rate Transition9/1
  Target_XY_Distance/1(Target_Y_Distance_mux) -> Abs/1, Target_XY_TimeToCollision/1(Target_Y_Distance)
  Abs/1 -> Compare To Lane_Width/2/1
  Relational Operator1/1 -> Logical Operator/2
  Compare To AEB_Distance_To_Collision_Brake/1 -> Logical Operator/1
  Delay/1 -> Switch/1
  Switch2/1 -> Delay1/1, "AEB_Brake_id "/2(Brake_Demand_mux), MinMax/1
  Rate Transition8/1 -> "AEB_Brake_id "/3(Target_id_mux)
  Product/1 -> Switch2/3
  Delay1/1 -> Product/2
  [Vehicle_Speed] -> Compare To Constant/1
  Compare To Constant/1 -> Data Type Conversion2/1
  Rate Transition7/1 -> Switch2/2
  Constant3/1 -> Switch2/1
  Compare To Zero3/1 -> Product/1
  Rate Limiter/1 -> Compare To Zero3/1
  Data Type Conversion2/1 -> Rate Limiter/1
  AEB_Trigger/1(AEB_Trigger) -> Switch/2, Mux2/1, Mux2/2
  Demux/3 -> Relational Operator/1, Detect Change/1, Rate Transition8/1
  Demux/1 -> Target_XY_Distance/1(Target_distance_mux)
  Demux/2 -> Target_XY_Distance/2(Target_azimuth_mux)
  Compare To Constant1/1 -> AEB_Trigger/1(In1)
  Rate Transition9/1 -> AEB_Trigger/5(In4)
  Compare To Lane_Width/2/1 -> AEB_Trigger/2(In5)
  Relational Operator/1 -> AEB_Trigger/4(In3)
  Logical Operator/1 -> Data Type Conversion1/1
  Target_XY_Distance/2(Target_X_Distance_mux) -> Target_XY_TimeToCollision/2(Target_X_Distance), Distance_To_Collision_computation/1(Distance), Compare To AEB_Distance_To_Collision_Brake/1, derivation_speed/1(Distance)
  [AEB_TimeToCollision_Threshold] -> Terminator/1
  Pulse Generator/1 -> derivation_speed/Trigger
  Rate Transition1/1 -> Compare To Constant1/1, Saturation/1
  derivation_speed/1(Speed_of_approaching) -> Rate Transition1/1
  filtering/1 -> Distance_To_Collision_computation/2(Speed)
  MATLAB Function/1(min_distance) -> [Minimum_distance]
  [Minimum_distance] -> To Workspace/1

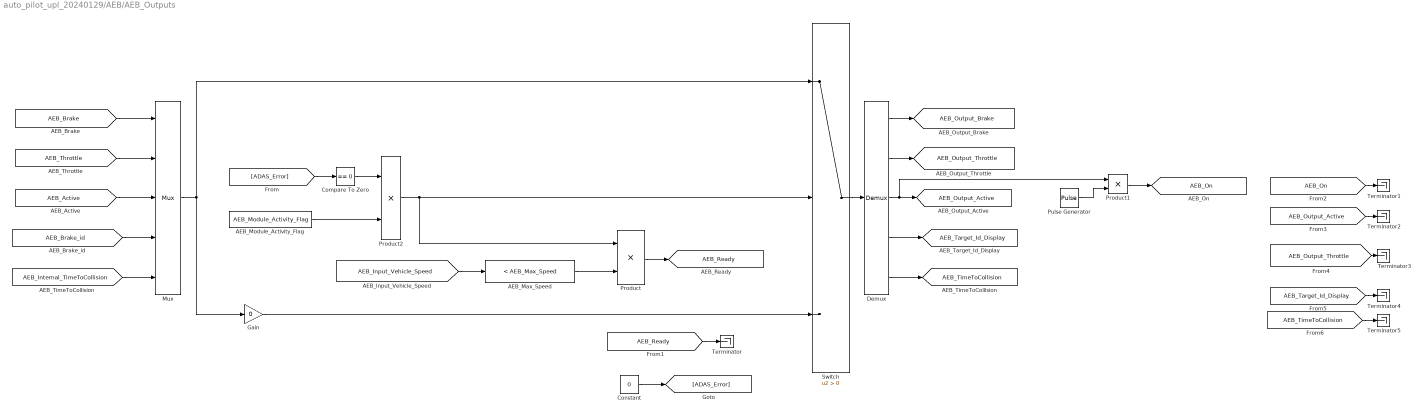
== system auto_pilot_upl_20240129/AEB/AEB_Outputs ==
  AEB_Max_Speed : simulink/Logic and Bit Operations/Compare To Constant  relop=<  const=AEB_Max_Speed  OutDataTypeStr=boolean
  AEB_Module_Activity_Flag : Constant  Value=AEB_Module_Activity_Flag
  Compare To Zero : simulink/Logic and Bit Operations/Compare To Zero  relop===  OutDataTypeStr=boolean
  Constant : Constant  Value=0
  Demux : Demux  Outputs=5
  Gain : Gain  Gain=0
  Mux : Mux  Inputs=5
  Product : Product
  Product1 : Product
  Product2 : Product
  Pulse Generator : DiscretePulseGenerator  PulseType=Time based  Period=1/AEB_Alarm_Freq  PulseWidth=50
  Switch : Switch  Criteria=u2 > Threshold  SaturateOnIntegerOverflow=off  InputSameDT=off
  Terminator{,1..5} (6 alike) : Terminator
  tag scope: AEB_On=global, AEB_Output_Active=global, AEB_Output_Brake=global, AEB_Output_Throttle=global, AEB_Ready=global, AEB_Target_Id_Display=global, AEB_TimeToCollision=global
  wires:
  [AEB_Brake] -> Mux/1
  [AEB_Throttle] -> Mux/2
  Mux/1 -> Switch/1, Gain/1
  Switch/1 -> Demux/1
  AEB_Module_Activity_Flag/1 -> Product2/2
  Demux/1 -> [AEB_Output_Brake]
  Demux/2 -> [AEB_Output_Throttle]
  Gain/1 -> Switch/3
  Demux/3 -> Product1/1, [AEB_Output_Active]
  [AEB_Active] -> Mux/3
  [AEB_Brake_id] -> Mux/4
  Demux/4 -> [AEB_Target_Id_Display]
  [AEB_Internal_TimeToCollision] -> Mux/5
  Demux/5 -> [AEB_TimeToCollision]
  [AEB_Input_Vehicle_Speed] -> AEB_Max_Speed/1
  AEB_Max_Speed/1 -> Product/2
  Pulse Generator/1 -> Product1/2
  [ADAS_Error] -> Compare To Zero/1
  Product2/1 -> Product/1, Switch/2
  Compare To Zero/1 -> Product2/1
  Product/1 -> [AEB_Ready]
  Product1/1 -> [AEB_On]
  [AEB_Ready] -> Terminator/1
  Constant/1 -> [ADAS_Error]
  [AEB_On] -> Terminator1/1
  [AEB_Output_Active] -> Terminator2/1
  [AEB_Output_Throttle] -> Terminator3/1
  [AEB_Target_Id_Display] -> Terminator4/1
  [AEB_TimeToCollision] -> Terminator5/1

== system auto_pilot_upl_20240129/AP/AP_Inputs ==
  Bus Creator : BusCreator  Inputs=2
  Demux : Demux  Outputs=2
  Gain4 : Gain  Gain=-1
  Mux4 : Mux  Inputs=2
  Terminator : Terminator
  tag scope: AP_Input_ACC_Ready=global, AP_Input_Driver_Brake=global, AP_Input_Driver_Steering=global, AP_Input_Driver_Throttle=global, AP_Input_LK_On_Request=global, AP_Input_laneGap_left=global, AP_Input_laneGap_right=global
  wires:
  [Driver_Steering] -> Gain4/1
  [mode] -> [AP_Input_LK_On_Request]
  [ACC_Ready] -> [AP_Input_ACC_Ready]
  [Driver_Brake] -> [AP_Input_Driver_Brake]
  [Driver_Throttle] -> [AP_Input_Driver_Throttle]
  [LaneGap_left_ws] -> Mux4/1
  Mux4/1 -> Demux/1
  [LaneGap_right_ws] -> Mux4/2
  Demux/1 -> [AP_Input_laneGap_left]
  Demux/2 -> [AP_Input_laneGap_right]
  Gain4/1 -> [AP_Input_Driver_Steering]
  [AP_Input_Driver_Brake] -> Bus Creator/1
  [AP_Input_Driver_Throttle] -> Bus Creator/2
  Bus Creator/1 -> Terminator/1
